simulink model "subsys_cont"  (R2018a)
settings: Solver=VariableStepAuto  StartTime=0.0  StopTime=10.0  RelTol=1e-3
libraries: dspsrcs4 x3
settings Model: Creator=Administrator  LastModifiedBy=Administrator

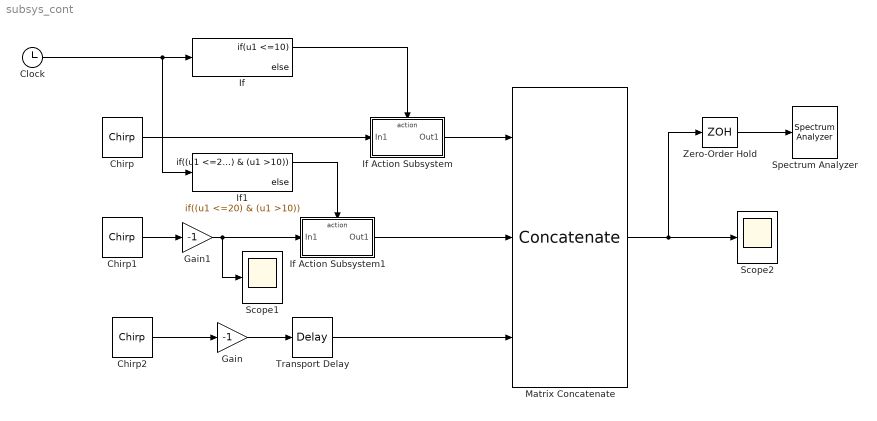
== system subsys_cont ==
  Chirp : dspsrcs4/Chirp  sweep=Logarithmic  mode=Unidirectional  f0=1000  f1=4000  t1=1  Tsweep=1  phase=0  Ts=1/1e6  spf=1  datatype=Double  OutputFrames=off
      settings: SourceProductName=DSP System Toolbox
  Chirp1 : dspsrcs4/Chirp  sweep=Logarithmic  mode=Unidirectional  f0=1000  f1=4000  t1=1  Tsweep=1  phase=0  Ts=1/1e6  spf=1  datatype=Double  OutputFrames=off
      settings: SourceProductName=DSP System Toolbox
  Chirp2 : dspsrcs4/Chirp  sweep=Logarithmic  mode=Unidirectional  f0=1000  f1=4000  t1=1  Tsweep=1  phase=0  Ts=1/1e6  spf=1  datatype=Double  OutputFrames=off
      settings: SourceProductName=DSP System Toolbox
  Clock : Clock
  Gain : Gain  Gain=-1
  Gain1 : Gain  Gain=-1
  If : If  IfExpression=u1 <=10
  If Action Subsystem : Subsystem  TreatAsAtomicUnit=on
  If Action Subsystem1 : Subsystem  TreatAsAtomicUnit=on
  If1 : If  IfExpression=(u1 <=20) & (u1 >10)
  Matrix Concatenate : Concatenate  NumInputs=3  Mode=Multidimensional array
  Scope1 : Scope
  Scope2 : Scope
  Spectrum Analyzer : SpectrumAnalyzer
  Transport Delay : TransportDelay  DelayTime=20
  Zero-Order Hold : ZeroOrderHold  SampleTime=-1
  wires:
  Chirp2/1 -> Gain/1
  If Action Subsystem/1(Out1) -> Matrix Concatenate/1
  If Action Subsystem1/1(Out1) -> Matrix Concatenate/2
  Chirp/1 -> If Action Subsystem/1(In1)
  Gain/1 -> Transport Delay/1
  If/1 -> If Action Subsystem/Action
  Chirp1/1 -> Gain1/1
  Matrix Concatenate/1 -> Zero-Order Hold/1, Scope2/1
  Gain1/1 -> Scope1/1, If Action Subsystem1/1(In1)
  Transport Delay/1 -> Matrix Concatenate/3
  If1/1 -> If Action Subsystem1/Action
  Clock/1 -> If1/1, If/1
  Zero-Order Hold/1 -> Spectrum Analyzer/1

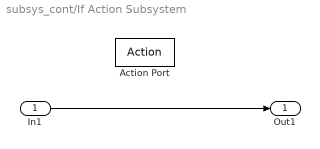
== system subsys_cont/If Action Subsystem ==
  In1 : Inport
  Action Port : ActionPort  ActionType=then
  Out1 : Outport
  wires:
  In1/1 -> Out1/1

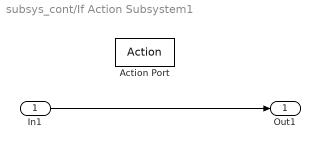
== system subsys_cont/If Action Subsystem1 ==
  In1 : Inport
  Action Port : ActionPort  ActionType=then
  Out1 : Outport
  wires:
  In1/1 -> Out1/1
